simulink model "bh_model_3FB"  (R2023a)
settings: Solver=daessc  StartTime=0.0  StopTime=100  MaxStep=0.005  RelTol=1e-4  AbsTol=1e-4  EnableMultiTasking=on
undefined symbols (not defined in the file or in its folder): env, P0, P1, P2, PA, PB, PC, PG, Points, Springs, Theta, W, X, Y, Z
libraries: sm_lib x34, nesl_utility x17
settings Model: Creator=bhorton  LastModifiedBy=bhorton
settings SolverCC: AutoScaleAbsTol=off  ZeroCrossAlgorithm=Adaptive  AlgebraicLoopSolver=TrustRegion  MaxZcPerStep=1
settings DataIOCC: LimitDataPoints=on  MaxDataPoints=10000  SaveOutput=off  SignalLogging=off  DSMLogging=off  SignalLoggingName=sigout  ReturnWorkspaceOutputsName=SIM_LOG_DATA
settings OptimizationCC: ReuseModelBlockBuffer=off  LifeSpan=inf
settings DebuggingCC: UnconnectedInputMsg=warning  UnconnectedOutputMsg=warning  UnconnectedLineMsg=warning  AllowSymbolicDim=off  SFUnexpectedBacktrackingDiag=warning  SFNoUnconditionalDefaultTransitionDiag=warning  SFExecutionAtInitializationDiag=none  ArithmeticOperatorsInVariantConditions=warning
settings ModelReferenceCC: EnableRefExpFcnMdlSchedulingChecks=on
settings SFSimCC: SimUseLocalCustomCode=off  CustomCodeUndefinedFunction=UseInterfaceOnly
settings RTWCC: RTWUseLocalCustomCode=off  DLArmComputeVersion=19.05
settings CodeAppCC: StateflowObjectComments=on
settings GRTTargetCC: TargetLangStandard=C89/C90 (ANSI)
settings ConfigComp: CovMetricSettings=dw  CovSaveCumulativeToWorkspaceVar=on  CovSaveSingleToWorkspaceVar=on  CovExternalEMLEnable=off  CovSFcnEnable=off
settings SimscapeCC: SimscapeLogType=all  SimscapeLogSimulationStatistics=on  SimscapeLogDataHistory=10000
settings ExplorerConfigSet: InternalSimMechanicsExplorerSettings="<ExplorerConfiguration><canonicalview>default</canonicalview><AnimationSetting><BasePlaybackSpeed>1.0</BasePlaybackSpeed><PlaybackSpeedFactor>1.0</PlaybackSpeedFactor></AnimationSetting><TilePanel><TileInfo><Tiles Columns=\"2\" Count=\"2\" Rows=\"1\"><Column Weight=\"0.4996\"/><Column Weight=\"0.5004\"/><Row Weight=\"1\"/><Tile Height=\"1\" Width=\"1\" X=\"0\" Y=\"0\"/><Tile Height=\"1\" Width=\"1\" X=\"1\" Y=\"0\"/></Tiles></TileInfo><SceneInfo><SceneViewer><BGColor><R>0.60000002384185791</R><G>0.60000002384185791</G><B>0.60000002384185791</B></BGColor><Camera><DoPerspective>off</DoPerspective><Position><X>0.491983639676432549</X><Y>0.660324737193826783</Y><Z>0.997500000159727507</Z></Position><Center><X>0.491983639676432549</X><Y>0.660324737193826783</Y><Z>-0.00249999984027249322</Z></Center><Up><X>0</X><Y>1</Y><Z>-0</Z></Up><ViewLimDist>1</ViewLimDist><YLim>0.930287200234285461</YLim><XLim>0.682141395707506204</XLim></Camera></SceneViewer><SceneViewer><BGColor><R>0.60000002384185791</R><G>0.60000002384185791</G><B>0.60000002384185791</B></BGColor><Camera><DoPerspective>off</DoPerspective><Position><X>0.536343126805734594</X><Y>1.50090638188909886</Y><Z>-0.103056785946452484</Z></Position><Center><X>0.536343126805734594</X><Y>0.499999971795685338</Y><Z>-0.103056785946452484</Z></Center><Up><X>0</X><Y>0</Y><Z>1</Z></Up><ViewLimDist>1</ViewLimDist><YLim>0.956987902738208662</YLim><XLim>0.702787991073371976</XLim></Camera></SceneViewer></SceneInfo></TilePanel><MechEditorPanel><Cameras/><GfxPanelCameraMap/><VideoCreator><PlaybackSpeedRatio>1.0</PlaybackSpeedRatio><FrameRate>30</FrameRate><VideoFormat>Motion JPEG AVI</VideoFormat><FrameSize>auto</FrameSize></VideoCreator></MechEditorPanel></ExplorerConfiguration>"

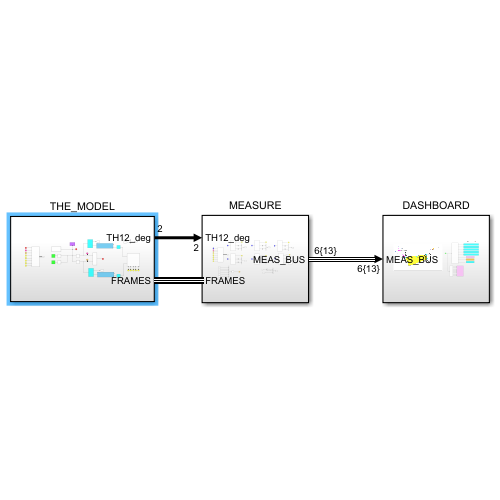
[thumbnail: Simulink's stored preview of the top-level diagram]
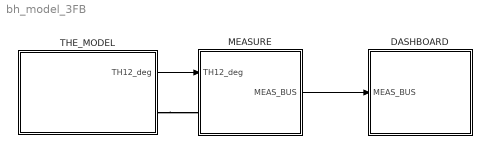
== system bh_model_3FB ==
  DASHBOARD : Subsystem
  MEASURE : Subsystem
  THE_MODEL : Subsystem
      settings: PortSchema="{\"entries\":[{\"content\":{\"sides\":[{\"content\":{\"connectorIds\":[\"Out1\",\"LConn1\"]},\"type\":\"ConnectorPlacement.EquallySpacedRectSide\",\"uuid\":\"a6bd5fb9-d314-4c72-8b76-e48d80fdb19b\"},{\"content\":{\"connectorIds\":[],\"side\":\"RIGHT\"},\"type\":\"ConnectorPlacement.EquallySpacedRectSide\",\"uuid\":\"36a13618-f0d5-425f-9c20-8177aa5c1d72\"},{\"content\":{\"connectorIds\":[],\"side\":\"TOP\"},\"type\":\"ConnectorPlacement.EquallySpacedRectSide\",\"uuid\":\"5c1dc12f-dfae-4687-beb7-ca64844c31e7\"}]},\"type\":\"ConnectorPlacement.EquallySpacedConnector\",\"uuid\":\"dc42e3a7-d8d3-4cef-9db1-f374fadbd399\"}],\"packageUris\":[\"http://schema.mathworks.com/mf0/Connector/R2020b\"],\"version\":\"1.0\"}"
  wires:
  THE_MODEL/1(TH12_deg) -> MEASURE/1(TH12_deg)
  MEASURE/1(MEAS_BUS) -> DASHBOARD/1(MEAS_BUS)
  connections:
  THE_MODEL/LConn1 -- MEASURE/LConn1

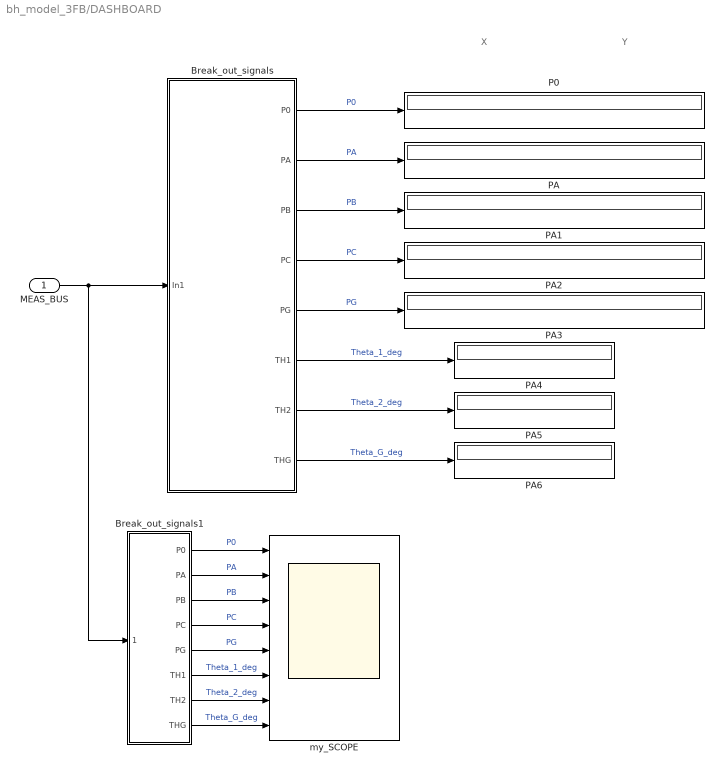
== system bh_model_3FB/DASHBOARD ==
  note: X
  note: Y
  MEAS_BUS : Inport
  Break_out_signals : Subsystem
  Break_out_signals1 : Subsystem
  P0 : Display
  PA{,1..6} (7 alike) : Display
  my_SCOPE : Scope  NumInputPorts=8
  wires:
  MEAS_BUS/1 -> Break_out_signals1/1(MEAS_BUS), Break_out_signals/1(In1)
  Break_out_signals/1(P0) -> P0/1  "P0"
  Break_out_signals/2(PA) -> PA/1  "PA"
  Break_out_signals/3(PB) -> PA1/1  "PB"
  Break_out_signals/4(PC) -> PA2/1  "PC"
  Break_out_signals/5(PG) -> PA3/1  "PG"
  Break_out_signals/6(TH1) -> PA4/1  "Theta_1_deg"
  Break_out_signals/7(TH2) -> PA5/1  "Theta_2_deg"
  Break_out_signals/8(THG) -> PA6/1  "Theta_G_deg"
  Break_out_signals1/1(P0) -> my_SCOPE/1  "P0"
  Break_out_signals1/2(PA) -> my_SCOPE/2  "PA"
  Break_out_signals1/3(PB) -> my_SCOPE/3  "PB"
  Break_out_signals1/4(PC) -> my_SCOPE/4  "PC"
  Break_out_signals1/5(PG) -> my_SCOPE/5  "PG"
  Break_out_signals1/6(TH1) -> my_SCOPE/6  "Theta_1_deg"
  Break_out_signals1/7(TH2) -> my_SCOPE/7  "Theta_2_deg"
  Break_out_signals1/8(THG) -> my_SCOPE/8  "Theta_G_deg"

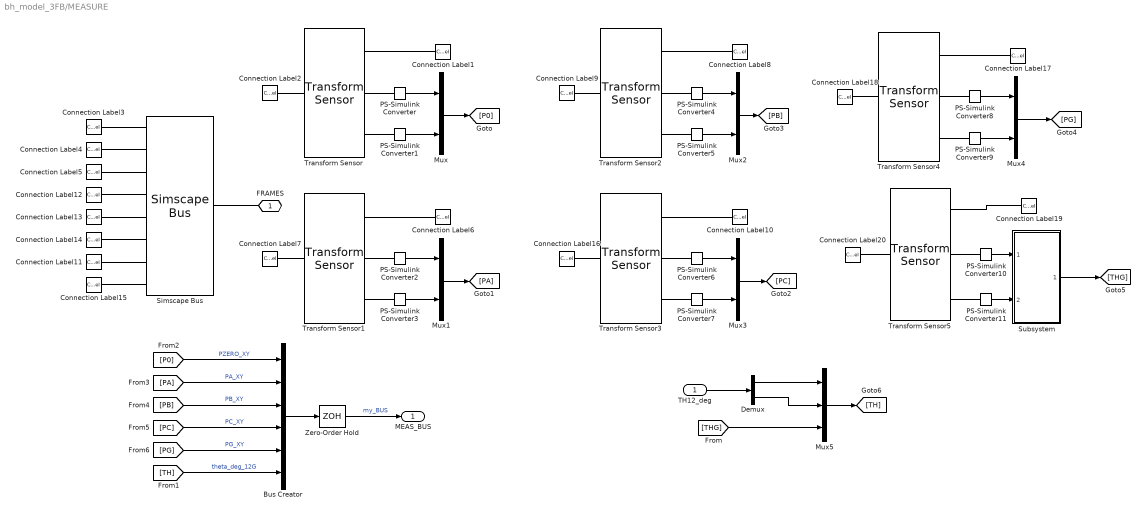
== system bh_model_3FB/MEASURE ==
  TH12_deg : Inport
  Bus Creator : BusCreator  Inputs=6
  Connection Label1 : ConnectionLabel  Label=P0
  Connection Label10 : ConnectionLabel  Label=PC
  Connection Label11 : ConnectionLabel  Label=P0
  Connection Label12 : ConnectionLabel  Label=PA
  Connection Label13 : ConnectionLabel  Label=PB
  Connection Label14 : ConnectionLabel  Label=PC
  Connection Label15 : ConnectionLabel  Label=PG
  Connection Label{2..3,7,9,16,18,20} (7 alike) : ConnectionLabel  Label=W
  Connection Label17 : ConnectionLabel  Label=PG
  Connection Label19 : ConnectionLabel  Label=PG
  Connection Label4 : ConnectionLabel  Label=P1
  Connection Label5 : ConnectionLabel  Label=P2
  Connection Label6 : ConnectionLabel  Label=PA
  Connection Label8 : ConnectionLabel  Label=PB
  Demux : Demux  Outputs=2
  Mux{,1..4} (5 alike) : Mux  Inputs=2
  Mux5 : Mux  Inputs=3
  PS-Simulink Converter{,1..9} (10 alike) : nesl_utility/PS-Simulink Converter  PhysicalDomain=network_engine_domain  SubClassName=ps_output  LeftPortType=input  RightPortType=output  PseudoPeriodic=off  Frequencies=[]  VectorFormat=inherit  Unit=m  AffineConversion=off
  PS-Simulink Converter10 : nesl_utility/PS-Simulink Converter  PhysicalDomain=network_engine_domain  SubClassName=ps_output  LeftPortType=input  RightPortType=output  PseudoPeriodic=off  Frequencies=[]  VectorFormat=inherit  Unit=deg  AffineConversion=off
  PS-Simulink Converter11 : nesl_utility/PS-Simulink Converter  PhysicalDomain=network_engine_domain  SubClassName=ps_output  LeftPortType=input  RightPortType=output  PseudoPeriodic=off  Frequencies=[]  VectorFormat=inherit  Unit=1  AffineConversion=off
  Simscape Bus : SimscapeBus  HierarchyStrings=W;P1;P2;PA;PB;PC;P0;PG
  Subsystem : Subsystem
  Transform Sensor{,1..4} (5 alike) : sm_lib/Frames and Transforms/Transform Sensor  MeasurementFrame=Base  RotationSequence=XYX  SenseAngle=off  SenseAxis=off  SenseQ=off  SenseR=off  SenseRotationSequence=off  SenseOmegaX=off  SenseOmegaY=off  SenseOmegaZ=off  SenseQDot=off  SenseRDot=off  SenseRotationSequenceDot=off  SenseAlphaX=off  SenseAlphaY=off  SenseAlphaZ=off  SenseQDDot=off  SenseRDDot=off  SenseX=on  SenseY=on  SenseZ=off  SenseRad=off  SenseAzim=off  SenseDist=off  SenseInc=off  SenseXDot=off  SenseYDot=off  SenseZDot=off  SenseRadDot=off  SenseAzimDot=off  SenseDistDot=off  SenseIncDot=off  SenseXDDot=off  SenseYDDot=off  SenseZDDot=off  SenseRadDDot=off  SenseAzimDDot=off  SenseDistDDot=off  SenseIncDDot=off
  Transform Sensor5 : sm_lib/Frames and Transforms/Transform Sensor  MeasurementFrame=Base  RotationSequence=XYX  SenseAngle=on  SenseAxis=on  SenseQ=off  SenseR=off  SenseRotationSequence=off  SenseOmegaX=off  SenseOmegaY=off  SenseOmegaZ=off  SenseQDot=off  SenseRDot=off  SenseRotationSequenceDot=off  SenseAlphaX=off  SenseAlphaY=off  SenseAlphaZ=off  SenseQDDot=off  SenseRDDot=off  SenseX=off  SenseY=off  SenseZ=off  SenseRad=off  SenseAzim=off  SenseDist=off  SenseInc=off  SenseXDot=off  SenseYDot=off  SenseZDot=off  SenseRadDot=off  SenseAzimDot=off  SenseDistDot=off  SenseIncDot=off  SenseXDDot=off  SenseYDDot=off  SenseZDDot=off  SenseRadDDot=off  SenseAzimDDot=off  SenseDistDDot=off  SenseIncDDot=off
  Zero-Order Hold : ZeroOrderHold  SampleTime=0.01
  FRAMES : PMIOPort  Side=Left
  MEAS_BUS : Outport
  wires:
  PS-Simulink Converter/1 -> Mux/1
  PS-Simulink Converter1/1 -> Mux/2
  PS-Simulink Converter3/1 -> Mux1/2
  PS-Simulink Converter2/1 -> Mux1/1
  PS-Simulink Converter4/1 -> Mux2/1
  PS-Simulink Converter5/1 -> Mux2/2
  PS-Simulink Converter6/1 -> Mux3/1
  PS-Simulink Converter7/1 -> Mux3/2
  PS-Simulink Converter8/1 -> Mux4/1
  PS-Simulink Converter9/1 -> Mux4/2
  PS-Simulink Converter10/1 -> Subsystem/1(q_deg)
  PS-Simulink Converter11/1 -> Subsystem/2(q_axes)
  Mux/1 -> [P0]
  Mux1/1 -> [PA]
  Mux3/1 -> [PC]
  Mux2/1 -> [PB]
  Mux4/1 -> [PG]
  Subsystem/1(theta_deg) -> [THG]
  TH12_deg/1 -> Demux/1
  Demux/1 -> Mux5/1
  Demux/2 -> Mux5/2
  [THG] -> Mux5/3
  Mux5/1 -> [TH]
  [TH] -> Bus Creator/6  "theta_deg_12G"
  [P0] -> Bus Creator/1  "PZERO_XY"
  [PA] -> Bus Creator/2  "PA_XY"
  [PB] -> Bus Creator/3  "PB_XY"
  [PC] -> Bus Creator/4  "PC_XY"
  [PG] -> Bus Creator/5  "PG_XY"
  Bus Creator/1 -> Zero-Order Hold/1
  Zero-Order Hold/1 -> MEAS_BUS/1  "my_BUS"
  connections:
  Connection Label12/LConn1 -- Simscape Bus/LConn4
  Connection Label13/LConn1 -- Simscape Bus/LConn5
  FRAMES/RConn1 -- Simscape Bus/RConn1
  Connection Label15/LConn1 -- Simscape Bus/LConn8
  Connection Label11/LConn1 -- Simscape Bus/LConn7
  Connection Label4/LConn1 -- Simscape Bus/LConn2
  Connection Label3/LConn1 -- Simscape Bus/LConn1
  Connection Label5/LConn1 -- Simscape Bus/LConn3
  Connection Label14/LConn1 -- Simscape Bus/LConn6
  Connection Label1/LConn1 -- Transform Sensor/RConn1
  PS-Simulink Converter/LConn1 -- Transform Sensor/RConn2
  PS-Simulink Converter1/LConn1 -- Transform Sensor/RConn3
  Connection Label2/LConn1 -- Transform Sensor/LConn1
  Connection Label6/LConn1 -- Transform Sensor1/RConn1
  PS-Simulink Converter2/LConn1 -- Transform Sensor1/RConn2
  PS-Simulink Converter3/LConn1 -- Transform Sensor1/RConn3
  Connection Label7/LConn1 -- Transform Sensor1/LConn1
  Connection Label8/LConn1 -- Transform Sensor2/RConn1
  PS-Simulink Converter5/LConn1 -- Transform Sensor2/RConn3
  Connection Label9/LConn1 -- Transform Sensor2/LConn1
  PS-Simulink Converter4/LConn1 -- Transform Sensor2/RConn2
  PS-Simulink Converter6/LConn1 -- Transform Sensor3/RConn2
  Connection Label10/LConn1 -- Transform Sensor3/RConn1
  PS-Simulink Converter7/LConn1 -- Transform Sensor3/RConn3
  Connection Label16/LConn1 -- Transform Sensor3/LConn1
  PS-Simulink Converter9/LConn1 -- Transform Sensor4/RConn3
  PS-Simulink Converter8/LConn1 -- Transform Sensor4/RConn2
  Connection Label17/LConn1 -- Transform Sensor4/RConn1
  Connection Label18/LConn1 -- Transform Sensor4/LConn1
  Connection Label20/LConn1 -- Transform Sensor5/LConn1
  Connection Label19/LConn1 -- Transform Sensor5/RConn1
  PS-Simulink Converter11/LConn1 -- Transform Sensor5/RConn3
  PS-Simulink Converter10/LConn1 -- Transform Sensor5/RConn2

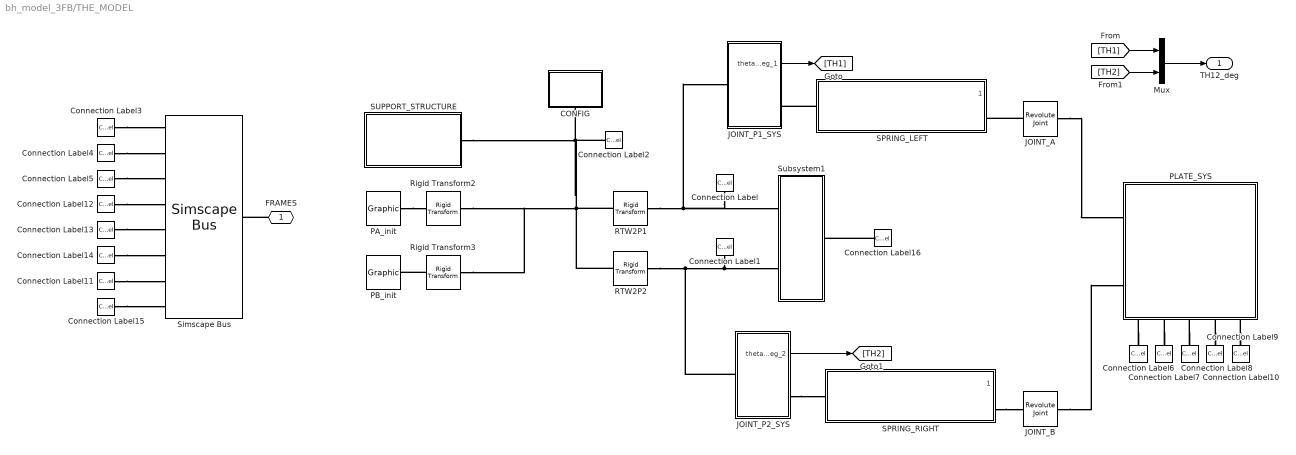
== system bh_model_3FB/THE_MODEL ==
  CONFIG : Subsystem
  Connection Label : ConnectionLabel  Label=P1
  Connection Label1 : ConnectionLabel  Label=P2
  Connection Label10 : ConnectionLabel  Label=P0
  Connection Label11 : ConnectionLabel  Label=P0
  Connection Label12 : ConnectionLabel  Label=PA
  Connection Label13 : ConnectionLabel  Label=PB
  Connection Label14 : ConnectionLabel  Label=PC
  Connection Label15 : ConnectionLabel  Label=PG
  Connection Label16 : ConnectionLabel  Label=W
  Connection Label2 : ConnectionLabel  Label=W
  Connection Label3 : ConnectionLabel  Label=W
  Connection Label4 : ConnectionLabel  Label=P1
  Connection Label5 : ConnectionLabel  Label=P2
  Connection Label6 : ConnectionLabel  Label=PA
  Connection Label7 : ConnectionLabel  Label=PB
  Connection Label8 : ConnectionLabel  Label=PC
  Connection Label9 : ConnectionLabel  Label=PG
  JOINT_A : sm_lib/Joints/Revolute Joint  JointMode=Normal  SenseConstraintForce=off  SenseConstraintForceX=off  SenseConstraintForceY=off  SenseConstraintForceZ=off  SenseConstraintTorque=off  SenseConstraintTorqueX=off  SenseConstraintTorqueY=off  SenseConstraintTorqueZ=off  SenseTotalForce=off  SenseTotalForceX=off  SenseTotalForceY=off  SenseTotalForceZ=off  SenseTotalTorque=off  SenseTotalTorqueX=off  SenseTotalTorqueY=off  SenseTotalTorqueZ=off  CompositeWrenchDir=FollowerOnBase  CompositeWrenchFrame=BaseFrame  EquilibriumPosition=0  EquilibriumPositionUnits=deg  SpringStiffness=0  SpringStiffnessUnits=N*m/deg  DampingCoefficient=0  DampingCoefficientUnits=N*m/(deg/s)  TorqueActuationMode=NoTorque  MotionActuationMode=ComputedMotion  SensePosition=off  SenseVelocity=off  SenseAcceleration=off  SenseTorqueForce=off  SenseLowerLimitTorqueForce=off  SenseUpperLimitTorqueForce=off  LowerLimitSpecify=off  LowerLimitBound=-90  LowerLimitBoundUnits=deg  LowerLimitStiffness=1e4  LowerLimitStiffnessUnits=N*m/deg  LowerLimitDamping=10  LowerLimitDampingUnits=N*m/(deg/s)  LowerLimitTransitionRegionWidth=0.1  LowerLimitTransitionRegionWidthUnits=deg  UpperLimitSpecify=off  UpperLimitBound=90  UpperLimitBoundUnits=deg  UpperLimitStiffness=1e4  UpperLimitStiffnessUnits=N*m/deg  UpperLimitDamping=10  UpperLimitDampingUnits=N*m/(deg/s)  UpperLimitTransitionRegionWidth=0.1  UpperLimitTransitionRegionWidthUnits=deg  PositionTargetSpecify=off  PositionTargetPriority=High  PositionTargetValue=-1*Theta.A_deg  PositionTargetValueUnits=deg  VelocityTargetSpecify=off  VelocityTargetPriority=High  VelocityTargetValue=0  VelocityTargetValueUnits=deg/s
  JOINT_B : sm_lib/Joints/Revolute Joint  JointMode=Normal  SenseConstraintForce=off  SenseConstraintForceX=off  SenseConstraintForceY=off  SenseConstraintForceZ=off  SenseConstraintTorque=off  SenseConstraintTorqueX=off  SenseConstraintTorqueY=off  SenseConstraintTorqueZ=off  SenseTotalForce=off  SenseTotalForceX=off  SenseTotalForceY=off  SenseTotalForceZ=off  SenseTotalTorque=off  SenseTotalTorqueX=off  SenseTotalTorqueY=off  SenseTotalTorqueZ=off  CompositeWrenchDir=FollowerOnBase  CompositeWrenchFrame=BaseFrame  EquilibriumPosition=0  EquilibriumPositionUnits=deg  SpringStiffness=0  SpringStiffnessUnits=N*m/deg  DampingCoefficient=0  DampingCoefficientUnits=N*m/(deg/s)  TorqueActuationMode=NoTorque  MotionActuationMode=ComputedMotion  SensePosition=off  SenseVelocity=off  SenseAcceleration=off  SenseTorqueForce=off  SenseLowerLimitTorqueForce=off  SenseUpperLimitTorqueForce=off  LowerLimitSpecify=off  LowerLimitBound=-90  LowerLimitBoundUnits=deg  LowerLimitStiffness=1e4  LowerLimitStiffnessUnits=N*m/deg  LowerLimitDamping=10  LowerLimitDampingUnits=N*m/(deg/s)  LowerLimitTransitionRegionWidth=0.1  LowerLimitTransitionRegionWidthUnits=deg  UpperLimitSpecify=off  UpperLimitBound=90  UpperLimitBoundUnits=deg  UpperLimitStiffness=1e4  UpperLimitStiffnessUnits=N*m/deg  UpperLimitDamping=10  UpperLimitDampingUnits=N*m/(deg/s)  UpperLimitTransitionRegionWidth=0.1  UpperLimitTransitionRegionWidthUnits=deg  PositionTargetSpecify=off  PositionTargetPriority=High  PositionTargetValue=-1*Theta.B_deg  PositionTargetValueUnits=deg  VelocityTargetSpecify=off  VelocityTargetPriority=High  VelocityTargetValue=0  VelocityTargetValueUnits=deg/s
  JOINT_P1_SYS : Subsystem
  JOINT_P2_SYS : Subsystem
  Mux : Mux  Inputs=2
  PA_init : sm_lib/Body Elements/Graphic  GraphicType=Marker  MarkerShape=Frame  MarkerSize=25  GraphicVisPropType=SimpleVisualProperties  GraphicDiffuseColor=[0 1 0]  GraphicSpecularColor=[0.5 0.5 0.5 1.0]  GraphicAmbientColor=[0.15 0.15 0.15 1.0]  GraphicEmissiveColor=[0.0 0.0 0.0 1.0]  GraphicShininess=75  GraphicOpacity=1.0
  PB_init : sm_lib/Body Elements/Graphic  GraphicType=Marker  MarkerShape=Frame  MarkerSize=25  GraphicVisPropType=SimpleVisualProperties  GraphicDiffuseColor=[0 1 0]  GraphicSpecularColor=[0.5 0.5 0.5 1.0]  GraphicAmbientColor=[0.15 0.15 0.15 1.0]  GraphicEmissiveColor=[0.0 0.0 0.0 1.0]  GraphicShininess=75  GraphicOpacity=1.0
  PLATE_SYS : Subsystem
      settings: PortSchema="{\"entries\":[{\"content\":{\"sides\":[{\"content\":{\"connectorIds\":[\"LConn1\",\"LConn2\"]},\"type\":\"ConnectorPlacement.EquallySpacedRectSide\",\"uuid\":\"93248c55-1ad3-445b-b9a7-56eb06c57406\"},{\"content\":{\"connectorIds\":[],\"side\":\"RIGHT\"},\"type\":\"ConnectorPlacement.EquallySpacedRectSide\",\"uuid\":\"b10a17e2-6726-4405-a35d-9fd4ae8c4b56\"},{\"content\":{\"connectorIds\":[],\"side\":\"TOP\"},\"type\":\"ConnectorPlacement.EquallySpacedRectSide\",\"uuid\":\"5c823850-66f1-4a0f-a96b-d5e6f0dcea4f\"},{\"content\":{\"connectorIds\":[\"RConn1\",\"RConn2\",\"RConn3\",\"RConn4\",\"RConn5\"],\"side\":\"BOTTOM\"},\"type\":\"ConnectorPlacement.EquallySpacedRectSide\",\"uuid\":\"67c94115-9b67-4c68-a1df-5a4847aab27d\"}]},\"type\":\"ConnectorPlacement.EquallySpacedConnector\",\"uuid\":\"0a1a3765-94d9-4f20-8fe4-7302b2902fa4\"}],\"packageUris\":[\"http://schema.mathworks.com/mf0/Connector/R2020b\"],\"version\":\"1.0\"}"
  RTW2P1 : sm_lib/Frames and Transforms/Rigid Transform  TranslationMethod=Cartesian  TranslationStandardOffset=0  TranslationStandardOffsetUnits=m  TranslationStandardAxis=+Z  TranslationCartesianOffset=[Points.P1, 0]  TranslationCartesianOffsetUnits=m  TranslationROffset=0  TranslationROffsetUnits=m  TranslationZOffset=0  TranslationZOffsetUnits=m  TranslationThetaOffset=0  TranslationThetaOffsetUnits=deg  RotationMethod=None  RotationAngleUnits=deg  RotationStandardAxis=+Z  RotationAngle=0.0  RotationArbitraryAxis=[0 0 1]  FollAlignAxisA=+X  BaseAlignAxisA=+Y  FollAlignAxisB=+Y  BaseAlignAxisB=+Z  RotationSequenceAxes=FollowerAxes  RotationSequence=XYX  RotationSequenceAngles=[0 0 0]  RotationSequenceAnglesUnits=deg  RotationMatrix=[1 0 0; 0 1 0; 0 0 1]  Quaternion=[1 0 0 0]
  RTW2P2 : sm_lib/Frames and Transforms/Rigid Transform  TranslationMethod=Cartesian  TranslationStandardOffset=0  TranslationStandardOffsetUnits=m  TranslationStandardAxis=+Z  TranslationCartesianOffset=[Points.P2, 0]  TranslationCartesianOffsetUnits=m  TranslationROffset=0  TranslationROffsetUnits=m  TranslationZOffset=0  TranslationZOffsetUnits=m  TranslationThetaOffset=0  TranslationThetaOffsetUnits=deg  RotationMethod=None  RotationAngleUnits=deg  RotationStandardAxis=+Z  RotationAngle=0.0  RotationArbitraryAxis=[0 0 1]  FollAlignAxisA=+X  BaseAlignAxisA=+Y  FollAlignAxisB=+Y  BaseAlignAxisB=+Z  RotationSequenceAxes=FollowerAxes  RotationSequence=XYX  RotationSequenceAngles=[0 0 0]  RotationSequenceAnglesUnits=deg  RotationMatrix=[1 0 0; 0 1 0; 0 0 1]  Quaternion=[1 0 0 0]
  Rigid Transform2 : sm_lib/Frames and Transforms/Rigid Transform  TranslationMethod=Cartesian  TranslationStandardOffset=0  TranslationStandardOffsetUnits=m  TranslationStandardAxis=+Z  TranslationCartesianOffset=[Points.PA, 0]  TranslationCartesianOffsetUnits=m  TranslationROffset=0  TranslationROffsetUnits=m  TranslationZOffset=0  TranslationZOffsetUnits=m  TranslationThetaOffset=0  TranslationThetaOffsetUnits=deg  RotationMethod=None  RotationAngleUnits=deg  RotationStandardAxis=+Z  RotationAngle=0.0  RotationArbitraryAxis=[0 0 1]  FollAlignAxisA=+X  BaseAlignAxisA=+Y  FollAlignAxisB=+Y  BaseAlignAxisB=+Z  RotationSequenceAxes=FollowerAxes  RotationSequence=XYX  RotationSequenceAngles=[0 0 0]  RotationSequenceAnglesUnits=deg  RotationMatrix=[1 0 0; 0 1 0; 0 0 1]  Quaternion=[1 0 0 0]
  Rigid Transform3 : sm_lib/Frames and Transforms/Rigid Transform  TranslationMethod=Cartesian  TranslationStandardOffset=0  TranslationStandardOffsetUnits=m  TranslationStandardAxis=+Z  TranslationCartesianOffset=[Points.PB, 0]  TranslationCartesianOffsetUnits=m  TranslationROffset=0  TranslationROffsetUnits=m  TranslationZOffset=0  TranslationZOffsetUnits=m  TranslationThetaOffset=0  TranslationThetaOffsetUnits=deg  RotationMethod=None  RotationAngleUnits=deg  RotationStandardAxis=+Z  RotationAngle=0.0  RotationArbitraryAxis=[0 0 1]  FollAlignAxisA=+X  BaseAlignAxisA=+Y  FollAlignAxisB=+Y  BaseAlignAxisB=+Z  RotationSequenceAxes=FollowerAxes  RotationSequence=XYX  RotationSequenceAngles=[0 0 0]  RotationSequenceAnglesUnits=deg  RotationMatrix=[1 0 0; 0 1 0; 0 0 1]  Quaternion=[1 0 0 0]
  SPRING_LEFT : Subsystem  ReferencedSubsystem=bh_COMPONENT_spring_SYS  k=Springs.LEFT.stiffness  c=Springs.LEFT.damping  EQ_L=Springs.LEFT.free_length  tip_pos_L=Springs.LEFT.initial_length  VIS_L=Springs.LEFT.visual_length  VIS_R=Springs.LEFT.visual_R
  SPRING_RIGHT : Subsystem  ReferencedSubsystem=bh_COMPONENT_spring_SYS  k=Springs.RIGHT.stiffness  c=Springs.RIGHT.damping  EQ_L=Springs.RIGHT.free_length  tip_pos_L=Springs.RIGHT.initial_length  VIS_L=Springs.RIGHT.visual_length  VIS_R=Springs.RIGHT.visual_R
  SUPPORT_STRUCTURE : Subsystem
  Simscape Bus : SimscapeBus  HierarchyStrings=W;P1;P2;PA;PB;PC;P0;PG
  Subsystem1 : Subsystem
  FRAMES : PMIOPort  Side=Left
  TH12_deg : Outport
  wires:
  JOINT_P2_SYS/1(theta_deg_2) -> [TH2]
  JOINT_P1_SYS/1(theta_deg_1) -> [TH1]
  [TH1] -> Mux/1
  [TH2] -> Mux/2
  Mux/1 -> TH12_deg/1
  connections:
  Connection Label15/LConn1 -- Simscape Bus/LConn8
  Connection Label11/LConn1 -- Simscape Bus/LConn7
  FRAMES/RConn1 -- Simscape Bus/RConn1
  RTW2P2/LConn1 -- RTW2P1/LConn1 -- Rigid Transform3/LConn1 -- Rigid Transform2/LConn1 -- Connection Label2/LConn1 -- SUPPORT_STRUCTURE/LConn1 -- CONFIG/LConn1
  PA_init/RConn1 -- Rigid Transform2/RConn1
  JOINT_B/RConn1 -- PLATE_SYS/LConn2
  Connection Label4/LConn1 -- Simscape Bus/LConn2
  Connection Label9/LConn1 -- PLATE_SYS/RConn4
  Connection Label10/LConn1 -- PLATE_SYS/RConn5
  Rigid Transform3/RConn1 -- PB_init/RConn1
  Connection Label5/LConn1 -- Simscape Bus/LConn3
  JOINT_A/RConn1 -- PLATE_SYS/LConn1
  Connection Label7/LConn1 -- PLATE_SYS/RConn2
  Connection Label14/LConn1 -- Simscape Bus/LConn6
  Connection Label6/LConn1 -- PLATE_SYS/RConn1
  Connection Label8/LConn1 -- PLATE_SYS/RConn3
  Connection Label12/LConn1 -- Simscape Bus/LConn4
  Connection Label3/LConn1 -- Simscape Bus/LConn1
  JOINT_A/LConn1 -- SPRING_LEFT/RConn1
  Connection Label13/LConn1 -- Simscape Bus/LConn5
  Connection Label/LConn1 -- Subsystem1/RConn1 -- RTW2P1/RConn1 -- JOINT_P1_SYS/LConn1
  JOINT_P2_SYS/LConn1 -- Connection Label1/LConn1 -- Subsystem1/RConn2 -- RTW2P2/RConn1
  Connection Label16/LConn1 -- Subsystem1/LConn1
  SPRING_LEFT/LConn1 -- JOINT_P1_SYS/RConn1
  JOINT_P2_SYS/RConn1 -- SPRING_RIGHT/LConn1
  SPRING_RIGHT/RConn1 -- JOINT_B/LConn1

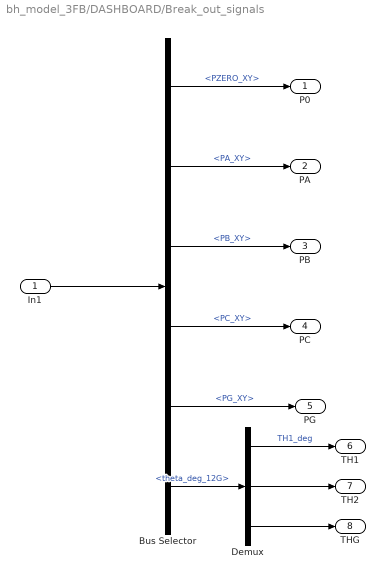
== system bh_model_3FB/DASHBOARD/Break_out_signals ==
  In1 : Inport
  Bus Selector : BusSelector  OutputSignals=PZERO_XY,PA_XY,PB_XY,PC_XY,PG_XY,theta_deg_12G
  Demux : Demux  Outputs=3
  P0 : Outport
  PA : Outport  Port=2
  PB : Outport  Port=3
  PC : Outport  Port=4
  PG : Outport  Port=5
  TH1 : Outport  Port=6
  TH2 : Outport  Port=7
  THG : Outport  Port=8
  wires:
  Demux/3 -> THG/1
  Bus Selector/3 -> PB/1  "<PB_XY>"
  Bus Selector/2 -> PA/1  "<PA_XY>"
  Bus Selector/5 -> PG/1  "<PG_XY>"
  Demux/1 -> TH1/1  "TH1_deg"
  Demux/2 -> TH2/1
  Bus Selector/6 -> Demux/1  "<theta_deg_12G>"
  Bus Selector/4 -> PC/1  "<PC_XY>"
  Bus Selector/1 -> P0/1  "<PZERO_XY>"
  In1/1 -> Bus Selector/1

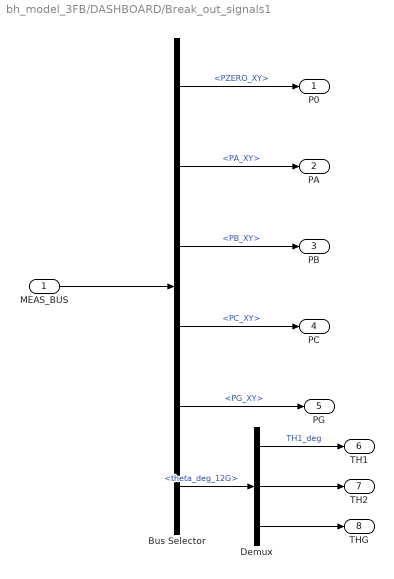
== system bh_model_3FB/DASHBOARD/Break_out_signals1 ==
  MEAS_BUS : Inport
  Bus Selector : BusSelector  OutputSignals=PZERO_XY,PA_XY,PB_XY,PC_XY,PG_XY,theta_deg_12G
  Demux : Demux  Outputs=3
  P0 : Outport
  PA : Outport  Port=2
  PB : Outport  Port=3
  PC : Outport  Port=4
  PG : Outport  Port=5
  TH1 : Outport  Port=6
  TH2 : Outport  Port=7
  THG : Outport  Port=8
  wires:
  Demux/3 -> THG/1
  Bus Selector/3 -> PB/1  "<PB_XY>"
  Bus Selector/2 -> PA/1  "<PA_XY>"
  Bus Selector/5 -> PG/1  "<PG_XY>"
  Demux/1 -> TH1/1  "TH1_deg"
  Demux/2 -> TH2/1
  Bus Selector/6 -> Demux/1  "<theta_deg_12G>"
  Bus Selector/4 -> PC/1  "<PC_XY>"
  Bus Selector/1 -> P0/1  "<PZERO_XY>"
  MEAS_BUS/1 -> Bus Selector/1

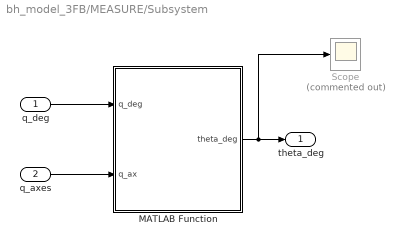
== system bh_model_3FB/MEASURE/Subsystem ==
  q_deg : Inport
  q_axes : Inport  Port=2
  MATLAB Function : MATLAB Function  TreatAsAtomicUnit=on
  Scope : Scope  Commented=on
  theta_deg : Outport
  wires:
  q_deg/1 -> MATLAB Function/1(q_deg)
  q_axes/1 -> MATLAB Function/2(q_ax)
  MATLAB Function/1(theta_deg) -> Scope/1, theta_deg/1

== system bh_model_3FB/THE_MODEL/CONFIG ==
  Mechanism Configuration : sm_lib/Utilities/Mechanism Configuration  UniformGravity=Constant  GravityVector=[0, -1*env.g, 0]  GravityVectorUnits=m/s^2  LinearizationDelta=0.001  JointModeTransitionNonlinearIterations=2
  Solver Configuration : nesl_utility/Solver Configuration  PhysicalDomain=network_engine_domain  SubClassName=solver  LeftPortType=input  RightPortType=generic  Tones=[]  Harmonics=[]  SimulateNoise=off  Profile=off  UseLocalSampling=off  EnableSwitchedLinearOptims=on  FrequencyDomain=off  UseCCode=off  RelTol=0.001  AbsTol=1e-06  MinStep=1e-09  ToWorkspace=off  RevertToSquareIcSolve=off  NumHomotopyIterations=100  PhasorMode=off  PhasorModeNumHarmonics=1  ConsistencySolver=NEWTON_FTOL  IndexReductionMethod=DerivativeReplacement  DoDC=off  ResidualTolerance=1e-09  ConsistencyTolSource=GLOBAL  ConsistencyAbsTol=0.001  ConsistencyRelTol=0.001  ConsistencyTolFactor=0.001  UseLocalSolver=off  LocalSolverChoice=NE_BACKWARD_EULER_ADVANCER  ResolveIndetEquations=on  FunctionEvalNumThread=1  LocalSolverSampleTime=0.001  DoFixedCost=off  MaxNonlinIter=3  MaxModeIter=2  ComputeImpulses=off  ImpulseIterations=2  LinearAlgebra=Sparse  LinearAlgebraNumThread=0  EquationFormulation=NE_TIME_EF  DelaysMemoryBudget=1024  AutomaticFiltering=on  FilteringTimeConstant=0.001  PartitionStorageMethod=AS_NEEDED  PartitionMemoryBudget=1024  PartitionMethod=FAST
  World Frame : sm_lib/Frames and Transforms/World Frame
  W : PMIOPort  Side=Left
  connections:
  World Frame/RConn1 -- Solver Configuration/RConn1 -- W/RConn1 -- Mechanism Configuration/RConn1

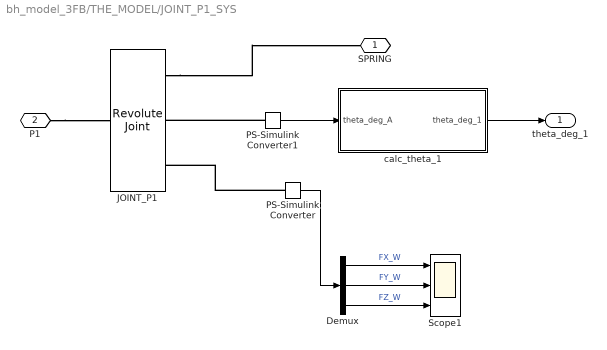
== system bh_model_3FB/THE_MODEL/JOINT_P1_SYS ==
  Demux : Demux  Outputs=3
  JOINT_P1 : sm_lib/Joints/Revolute Joint  JointMode=Normal  SenseConstraintForce=on  SenseConstraintForceX=off  SenseConstraintForceY=off  SenseConstraintForceZ=off  SenseConstraintTorque=off  SenseConstraintTorqueX=off  SenseConstraintTorqueY=off  SenseConstraintTorqueZ=off  SenseTotalForce=off  SenseTotalForceX=off  SenseTotalForceY=off  SenseTotalForceZ=off  SenseTotalTorque=off  SenseTotalTorqueX=off  SenseTotalTorqueY=off  SenseTotalTorqueZ=off  CompositeWrenchDir=BaseOnFollower  CompositeWrenchFrame=BaseFrame  EquilibriumPosition=0  EquilibriumPositionUnits=deg  SpringStiffness=0  SpringStiffnessUnits=N*m/deg  DampingCoefficient=0  DampingCoefficientUnits=N*m/(deg/s)  TorqueActuationMode=NoTorque  MotionActuationMode=ComputedMotion  SensePosition=on  SenseVelocity=off  SenseAcceleration=off  SenseTorqueForce=off  SenseLowerLimitTorqueForce=off  SenseUpperLimitTorqueForce=off  LowerLimitSpecify=off  LowerLimitBound=-90  LowerLimitBoundUnits=deg  LowerLimitStiffness=1e4  LowerLimitStiffnessUnits=N*m/deg  LowerLimitDamping=10  LowerLimitDampingUnits=N*m/(deg/s)  LowerLimitTransitionRegionWidth=0.1  LowerLimitTransitionRegionWidthUnits=deg  UpperLimitSpecify=off  UpperLimitBound=90  UpperLimitBoundUnits=deg  UpperLimitStiffness=1e4  UpperLimitStiffnessUnits=N*m/deg  UpperLimitDamping=10  UpperLimitDampingUnits=N*m/(deg/s)  UpperLimitTransitionRegionWidth=0.1  UpperLimitTransitionRegionWidthUnits=deg  PositionTargetSpecify=on  PositionTargetPriority=High  PositionTargetValue=Theta.A_deg  PositionTargetValueUnits=deg  VelocityTargetSpecify=on  VelocityTargetPriority=High  VelocityTargetValue=0  VelocityTargetValueUnits=deg/s
  PS-Simulink Converter : nesl_utility/PS-Simulink Converter  PhysicalDomain=network_engine_domain  SubClassName=ps_output  LeftPortType=input  RightPortType=output  PseudoPeriodic=off  Frequencies=[]  VectorFormat=inherit  Unit=N  AffineConversion=off
  PS-Simulink Converter1 : nesl_utility/PS-Simulink Converter  PhysicalDomain=network_engine_domain  SubClassName=ps_output  LeftPortType=input  RightPortType=output  PseudoPeriodic=off  Frequencies=[]  VectorFormat=inherit  Unit=deg  AffineConversion=off
  Scope1 : Scope  NumInputPorts=3
  calc_theta_1 : Subsystem
  SPRING : PMIOPort  Side=Right
  P1 : PMIOPort  Port=2  Side=Left
  theta_deg_1 : Outport
  wires:
  Demux/2 -> Scope1/2  "FY_W"
  PS-Simulink Converter/1 -> Demux/1
  Demux/1 -> Scope1/1  "FX_W"
  Demux/3 -> Scope1/3  "FZ_W"
  PS-Simulink Converter1/1 -> calc_theta_1/1(theta_deg_A)
  calc_theta_1/1(theta_deg_1) -> theta_deg_1/1
  connections:
  JOINT_P1/RConn1 -- SPRING/RConn1
  P1/RConn1 -- JOINT_P1/LConn1
  PS-Simulink Converter/LConn1 -- JOINT_P1/RConn3
  PS-Simulink Converter1/LConn1 -- JOINT_P1/RConn2

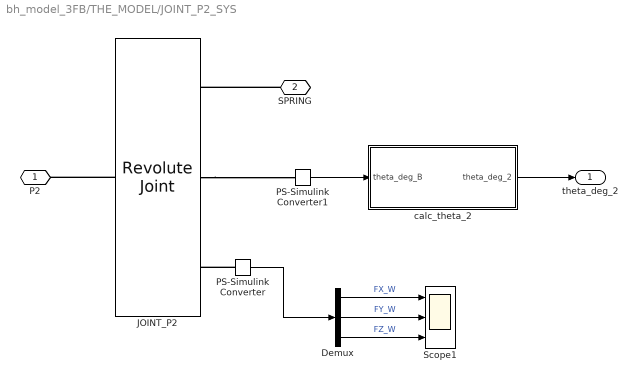
== system bh_model_3FB/THE_MODEL/JOINT_P2_SYS ==
  Demux : Demux  Outputs=3
  JOINT_P2 : sm_lib/Joints/Revolute Joint  JointMode=Normal  SenseConstraintForce=on  SenseConstraintForceX=off  SenseConstraintForceY=off  SenseConstraintForceZ=off  SenseConstraintTorque=off  SenseConstraintTorqueX=off  SenseConstraintTorqueY=off  SenseConstraintTorqueZ=off  SenseTotalForce=off  SenseTotalForceX=off  SenseTotalForceY=off  SenseTotalForceZ=off  SenseTotalTorque=off  SenseTotalTorqueX=off  SenseTotalTorqueY=off  SenseTotalTorqueZ=off  CompositeWrenchDir=FollowerOnBase  CompositeWrenchFrame=BaseFrame  EquilibriumPosition=0  EquilibriumPositionUnits=deg  SpringStiffness=0  SpringStiffnessUnits=N*m/deg  DampingCoefficient=0  DampingCoefficientUnits=N*m/(deg/s)  TorqueActuationMode=NoTorque  MotionActuationMode=ComputedMotion  SensePosition=on  SenseVelocity=off  SenseAcceleration=off  SenseTorqueForce=off  SenseLowerLimitTorqueForce=off  SenseUpperLimitTorqueForce=off  LowerLimitSpecify=off  LowerLimitBound=-90  LowerLimitBoundUnits=deg  LowerLimitStiffness=1e4  LowerLimitStiffnessUnits=N*m/deg  LowerLimitDamping=10  LowerLimitDampingUnits=N*m/(deg/s)  LowerLimitTransitionRegionWidth=0.1  LowerLimitTransitionRegionWidthUnits=deg  UpperLimitSpecify=off  UpperLimitBound=90  UpperLimitBoundUnits=deg  UpperLimitStiffness=1e4  UpperLimitStiffnessUnits=N*m/deg  UpperLimitDamping=10  UpperLimitDampingUnits=N*m/(deg/s)  UpperLimitTransitionRegionWidth=0.1  UpperLimitTransitionRegionWidthUnits=deg  PositionTargetSpecify=on  PositionTargetPriority=High  PositionTargetValue=Theta.B_deg  PositionTargetValueUnits=deg  VelocityTargetSpecify=on  VelocityTargetPriority=High  VelocityTargetValue=0  VelocityTargetValueUnits=deg/s
  PS-Simulink Converter : nesl_utility/PS-Simulink Converter  PhysicalDomain=network_engine_domain  SubClassName=ps_output  LeftPortType=input  RightPortType=output  PseudoPeriodic=off  Frequencies=[]  VectorFormat=inherit  Unit=N  AffineConversion=off
  PS-Simulink Converter1 : nesl_utility/PS-Simulink Converter  PhysicalDomain=network_engine_domain  SubClassName=ps_output  LeftPortType=input  RightPortType=output  PseudoPeriodic=off  Frequencies=[]  VectorFormat=inherit  Unit=deg  AffineConversion=off
  Scope1 : Scope  NumInputPorts=3
  calc_theta_2 : Subsystem
  P2 : PMIOPort  Side=Left
  SPRING : PMIOPort  Port=2  Side=Right
  theta_deg_2 : Outport
  wires:
  Demux/1 -> Scope1/1  "FX_W"
  Demux/3 -> Scope1/3  "FZ_W"
  Demux/2 -> Scope1/2  "FY_W"
  PS-Simulink Converter/1 -> Demux/1
  calc_theta_2/1(theta_deg_2) -> theta_deg_2/1
  PS-Simulink Converter1/1 -> calc_theta_2/1(theta_deg_B)
  connections:
  JOINT_P2/LConn1 -- P2/RConn1
  SPRING/RConn1 -- JOINT_P2/RConn1
  PS-Simulink Converter/LConn1 -- JOINT_P2/RConn3
  JOINT_P2/RConn2 -- PS-Simulink Converter1/LConn1

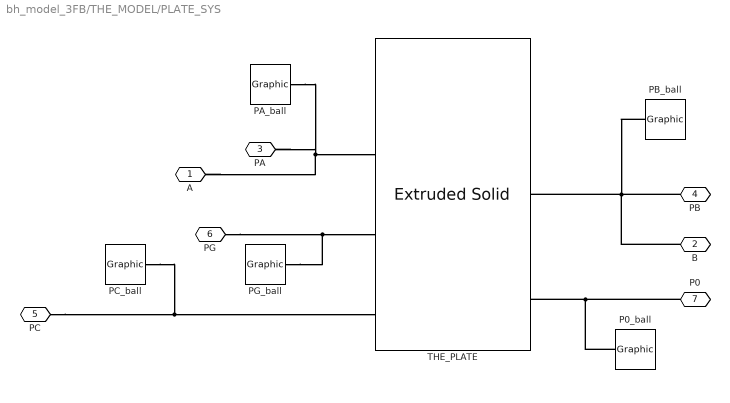
== system bh_model_3FB/THE_MODEL/PLATE_SYS ==
  P0_ball : sm_lib/Body Elements/Graphic  GraphicType=Marker  MarkerShape=Sphere  MarkerSize=10  GraphicVisPropType=SimpleVisualProperties  GraphicDiffuseColor=[0 1 1]  GraphicSpecularColor=[0.5 0.5 0.5 1.0]  GraphicAmbientColor=[0.15 0.15 0.15 1.0]  GraphicEmissiveColor=[0.0 0.0 0.0 1.0]  GraphicShininess=75  GraphicOpacity=1.0
  PA_ball : sm_lib/Body Elements/Graphic  GraphicType=Marker  MarkerShape=Sphere  MarkerSize=10  GraphicVisPropType=SimpleVisualProperties  GraphicDiffuseColor=[0 1 1]  GraphicSpecularColor=[0.5 0.5 0.5 1.0]  GraphicAmbientColor=[0.15 0.15 0.15 1.0]  GraphicEmissiveColor=[0.0 0.0 0.0 1.0]  GraphicShininess=75  GraphicOpacity=1.0
  PB_ball : sm_lib/Body Elements/Graphic  GraphicType=Marker  MarkerShape=Sphere  MarkerSize=10  GraphicVisPropType=SimpleVisualProperties  GraphicDiffuseColor=[0 1 1]  GraphicSpecularColor=[0.5 0.5 0.5 1.0]  GraphicAmbientColor=[0.15 0.15 0.15 1.0]  GraphicEmissiveColor=[0.0 0.0 0.0 1.0]  GraphicShininess=75  GraphicOpacity=1.0
  PC_ball : sm_lib/Body Elements/Graphic  GraphicType=Marker  MarkerShape=Sphere  MarkerSize=10  GraphicVisPropType=SimpleVisualProperties  GraphicDiffuseColor=[0 1 1]  GraphicSpecularColor=[0.5 0.5 0.5 1.0]  GraphicAmbientColor=[0.15 0.15 0.15 1.0]  GraphicEmissiveColor=[0.0 0.0 0.0 1.0]  GraphicShininess=75  GraphicOpacity=1.0
  PG_ball : sm_lib/Body Elements/Graphic  GraphicType=Marker  MarkerShape=Sphere  MarkerSize=10  GraphicVisPropType=SimpleVisualProperties  GraphicDiffuseColor=[0 1 1]  GraphicSpecularColor=[0.5 0.5 0.5 1.0]  GraphicAmbientColor=[0.15 0.15 0.15 1.0]  GraphicEmissiveColor=[0.0 0.0 0.0 1.0]  GraphicShininess=75  GraphicOpacity=1.0
  THE_PLATE : sm_lib/Body Elements/Extruded Solid  GraphicAmbientColor=[0.15 0.15 0.15 1.0]  BasedOnType=Density  CenterOfMass=[0 0 0]  CenterOfMassUnits=m  GraphicDiffuseColor=[1.0 1.0 0.0]  ExportConvexHullGeometry=off  ExtrusionCrossSection=quad_obj.get_xy  ExtrusionCrossSectionUnits=m  Density=quad_obj.density  DensityUnits=kg/m^3  DoExposeReferenceFrame=on  GraphicEmissiveColor=[0.0 0.0 0.0 1.0]  ExportEntireGeometry=off  ExtrusionLength=quad_obj.z_thick  ExtrusionLengthUnits=m  ExtrusionType=General  SerializedFrames=<Frames><Frame><Id>Frame1</Id><Value><Name>CoM</Name><Origin><Source>CenterOfMassFrame</Source><FeatureName></FeatureName></Origin><PrimaryAxis><DefinedDirection>+Z</DefinedDirection><Source>ReferenceFrame</Source><SourceDirection>+Z</SourceDirection><FeatureName></FeatureName></PrimaryAxis><SecondaryAxis><DefinedDirection>+X</DefinedDirection><Source>ReferenceFrame</Source><SourceDirection>+X</SourceDirection><FeatureName></FeatureName></SecondaryAxis></Value></Frame><Frame><Id>Frame2</Id><Value><Name>A</Name><Origin><Source>GeometricFeature</Source><FeatureName>top point 4</FeatureName></Origin><PrimaryAxis><DefinedDirection>+Z</DefinedDirection><Source>ReferenceFrame</Source><SourceDirection>+Z</SourceDirection><FeatureName></FeatureName></PrimaryAxis><SecondaryAxis><DefinedDirection>+X</DefinedDirection><Source>ReferenceFrame</Source><SourceDirection>+X</SourceDirection><FeatureName></FeatureName></SecondaryAxis></Value></Frame><Frame><Id>Frame3</Id><Value><Name>B</Name><Origin><Source>GeometricFeature</Source><FeatureName>top point 3</FeatureName></Origin><PrimaryAxis><DefinedDirection>+Z</DefinedDirection><Source>ReferenceFrame</Source><SourceDirection>+Z</SourceDirection><FeatureName></FeatureName></PrimaryAxis><SecondaryAxis><DefinedDirection>+X</DefinedDirection><Source>ReferenceFrame</Source><SourceDirection>+X</SourceDirection><FeatureName></FeatureName></SecondaryAxis></Value></Frame><Frame><Id>Frame4</Id><Value><Name>COM_face</Name><Origin><Source>GeometricFeature</Source><FeatureName>top surface</FeatureName></Origin><PrimaryAxis><DefinedDirection>+Z</DefinedDirection><Source>ReferenceFrame</Source><SourceDirection>+Z</SourceDirection><FeatureName></FeatureName></PrimaryAxis><SecondaryAxis><DefinedDirection>+X</DefinedDirection><Source>ReferenceFrame</Source><SourceDirection>+X</SourceDirection><FeatureName></FeatureName></SecondaryAxis></Value></Frame><Frame><Id>Frame5</Id><Value><Name>0</Name><Origin><Source>GeometricFeature</Source><FeatureName>top point 1</FeatureName></Origin><PrimaryAxis><DefinedDirection>+Z</DefinedDirection><Source>ReferenceFrame</Source><SourceDirection>+Z</SourceDirection><FeatureName></FeatureName></PrimaryAxis><SecondaryAxis><DefinedDirection>+X</DefinedDirection><Source>ReferenceFrame</Source><SourceDirection>+X</SourceDirection><FeatureName></FeatureName></SecondaryAxis></Value></Frame><Frame><Id>Frame6</Id><Value><Name>C</Name><Origin><Source>GeometricFeature</Source><FeatureName>top point 2</FeatureName></Origin><PrimaryAxis><DefinedDirection>+Z</DefinedDirection><Source>ReferenceFrame</Source><SourceDirection>+Z</SourceDirection><FeatureName></FeatureName></PrimaryAxis><SecondaryAxis><DefinedDirection>+X</DefinedDirection><Source>ReferenceFrame</Source><SourceDirection>+X</SourceDirection><FeatureName></FeatureName></SecondaryAxis></Value></Frame></Frames>  MarkerShape=Sphere  MarkerSize=10  GraphicType=FromGeometry  InertiaType=CalculateFromGeometry  Mass=1  MassUnits=kg  MomentsOfInertia=[1 1 1]  MomentsOfInertiaUnits=kg*m^2  PolygonNumSides=3  GraphicOpacity=1.0  PolygonOuterRadius=1  PolygonOuterRadiusUnits=m  ProductsOfInertia=[0 0 0]  ProductsOfInertiaUnits=kg*m^2  GraphicShininess=75  GraphicSpecularColor=[0.5 0.5 0.5 1.0]  GraphicVisPropType=SimpleVisualProperties
  A : PMIOPort  Side=Left
  B : PMIOPort  Port=2  Side=Left
  PA : PMIOPort  Port=3  Side=Right
  PB : PMIOPort  Port=4  Side=Right
  PC : PMIOPort  Port=5  Side=Right
  PG : PMIOPort  Port=6  Side=Right
  P0 : PMIOPort  Port=7  Side=Right
  connections:
  B/RConn1 -- PB_ball/RConn1 -- PB/RConn1 -- THE_PLATE/RConn2
  A/RConn1 -- PA_ball/RConn1 -- PA/RConn1 -- THE_PLATE/LConn2
  PG/RConn1 -- PG_ball/RConn1 -- THE_PLATE/LConn3
  PC/RConn1 -- THE_PLATE/LConn4 -- PC_ball/RConn1
  P0/RConn1 -- P0_ball/RConn1 -- THE_PLATE/RConn3

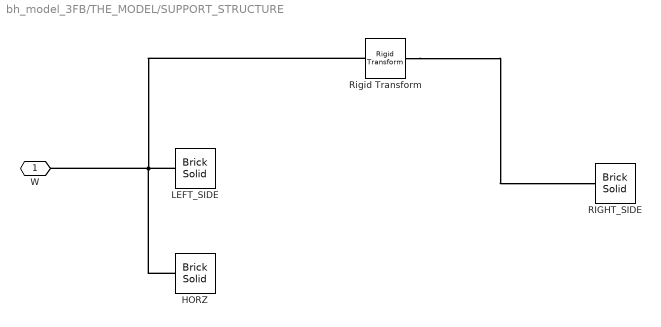
== system bh_model_3FB/THE_MODEL/SUPPORT_STRUCTURE ==
  HORZ : sm_lib/Body Elements/Brick Solid  GraphicAmbientColor=[0.15 0.15 0.15 1.0]  BasedOnType=Density  BrickDimensions=Support.HORZ.dims  BrickDimensionsUnits=m  CenterOfMass=[0 0 0]  CenterOfMassUnits=m  GraphicDiffuseColor=[0.0 0.0 0.0]  Density=1000  DensityUnits=kg/m^3  DoExposeReferenceFrame=on  GraphicEmissiveColor=[0.0 0.0 0.0 1.0]  ExportEntireGeometry=off  SerializedFrames=<Frames><Frame><Id>Frame1</Id><Value><Name>0</Name><Origin><Source>GeometricFeature</Source><FeatureName>+z -x curve</FeatureName></Origin><PrimaryAxis><DefinedDirection>+Z</DefinedDirection><Source>ReferenceFrame</Source><SourceDirection>+Z</SourceDirection><FeatureName></FeatureName></PrimaryAxis><SecondaryAxis><DefinedDirection>+X</DefinedDirection><Source>ReferenceFrame</Source><SourceDirection>+X</SourceDirection><FeatureName></FeatureName></SecondaryAxis></Value></Frame></Frames>  MarkerShape=Sphere  MarkerSize=10  GraphicType=FromGeometry  InertiaType=CalculateFromGeometry  Mass=1  MassUnits=kg  MomentsOfInertia=[1 1 1]  MomentsOfInertiaUnits=kg*m^2  GraphicOpacity=1.0  ProductsOfInertia=[0 0 0]  ProductsOfInertiaUnits=kg*m^2  GraphicShininess=75  GraphicSpecularColor=[0.5 0.5 0.5 1.0]  GraphicVisPropType=SimpleVisualProperties
  LEFT_SIDE : sm_lib/Body Elements/Brick Solid  GraphicAmbientColor=[0.15 0.15 0.15 1.0]  BasedOnType=Density  BrickDimensions=Support.VERT.dims  BrickDimensionsUnits=m  CenterOfMass=[0 0 0]  CenterOfMassUnits=m  GraphicDiffuseColor=[0.0 0.0 0.0]  Density=1000  DensityUnits=kg/m^3  DoExposeReferenceFrame=on  GraphicEmissiveColor=[0.0 0.0 0.0 1.0]  ExportEntireGeometry=off  SerializedFrames=<Frames><Frame><Id>Frame1</Id><Value><Name>0</Name><Origin><Source>GeometricFeature</Source><FeatureName>-y +z curve</FeatureName></Origin><PrimaryAxis><DefinedDirection>+Z</DefinedDirection><Source>ReferenceFrame</Source><SourceDirection>+Z</SourceDirection><FeatureName></FeatureName></PrimaryAxis><SecondaryAxis><DefinedDirection>+X</DefinedDirection><Source>ReferenceFrame</Source><SourceDirection>+X</SourceDirection><FeatureName></FeatureName></SecondaryAxis></Value></Frame></Frames>  MarkerShape=Sphere  MarkerSize=10  GraphicType=FromGeometry  InertiaType=CalculateFromGeometry  Mass=1  MassUnits=kg  MomentsOfInertia=[1 1 1]  MomentsOfInertiaUnits=kg*m^2  GraphicOpacity=1.0  ProductsOfInertia=[0 0 0]  ProductsOfInertiaUnits=kg*m^2  GraphicShininess=75  GraphicSpecularColor=[0.5 0.5 0.5 1.0]  GraphicVisPropType=SimpleVisualProperties
  RIGHT_SIDE : sm_lib/Body Elements/Brick Solid  GraphicAmbientColor=[0.15 0.15 0.15 1.0]  BasedOnType=Density  BrickDimensions=Support.VERT.dims  BrickDimensionsUnits=m  CenterOfMass=[0 0 0]  CenterOfMassUnits=m  GraphicDiffuseColor=[0.0 0.0 0.0]  Density=1000  DensityUnits=kg/m^3  DoExposeReferenceFrame=on  GraphicEmissiveColor=[0.0 0.0 0.0 1.0]  ExportEntireGeometry=off  SerializedFrames=<Frames><Frame><Id>Frame1</Id><Value><Name>0</Name><Origin><Source>GeometricFeature</Source><FeatureName>-y +z curve</FeatureName></Origin><PrimaryAxis><DefinedDirection>+Z</DefinedDirection><Source>ReferenceFrame</Source><SourceDirection>+Z</SourceDirection><FeatureName></FeatureName></PrimaryAxis><SecondaryAxis><DefinedDirection>+X</DefinedDirection><Source>ReferenceFrame</Source><SourceDirection>+X</SourceDirection><FeatureName></FeatureName></SecondaryAxis></Value></Frame></Frames>  MarkerShape=Sphere  MarkerSize=10  GraphicType=FromGeometry  InertiaType=CalculateFromGeometry  Mass=1  MassUnits=kg  MomentsOfInertia=[1 1 1]  MomentsOfInertiaUnits=kg*m^2  GraphicOpacity=1.0  ProductsOfInertia=[0 0 0]  ProductsOfInertiaUnits=kg*m^2  GraphicShininess=75  GraphicSpecularColor=[0.5 0.5 0.5 1.0]  GraphicVisPropType=SimpleVisualProperties
  Rigid Transform : sm_lib/Frames and Transforms/Rigid Transform  TranslationMethod=StandardAxis  TranslationStandardOffset=Points.P2(1)-Points.P1(1)  TranslationStandardOffsetUnits=m  TranslationStandardAxis=+X  TranslationCartesianOffset=[0 0 0]  TranslationCartesianOffsetUnits=m  TranslationROffset=0  TranslationROffsetUnits=m  TranslationZOffset=0  TranslationZOffsetUnits=m  TranslationThetaOffset=0  TranslationThetaOffsetUnits=deg  RotationMethod=None  RotationAngleUnits=deg  RotationStandardAxis=+Z  RotationAngle=0.0  RotationArbitraryAxis=[0 0 1]  FollAlignAxisA=+X  BaseAlignAxisA=+Y  FollAlignAxisB=+Y  BaseAlignAxisB=+Z  RotationSequenceAxes=FollowerAxes  RotationSequence=XYX  RotationSequenceAngles=[0 0 0]  RotationSequenceAnglesUnits=deg  RotationMatrix=[1 0 0; 0 1 0; 0 0 1]  Quaternion=[1 0 0 0]
  W : PMIOPort  Side=Left
  connections:
  LEFT_SIDE/LConn1 -- W/RConn1 -- Rigid Transform/LConn1 -- HORZ/LConn1
  Rigid Transform/RConn1 -- RIGHT_SIDE/LConn1

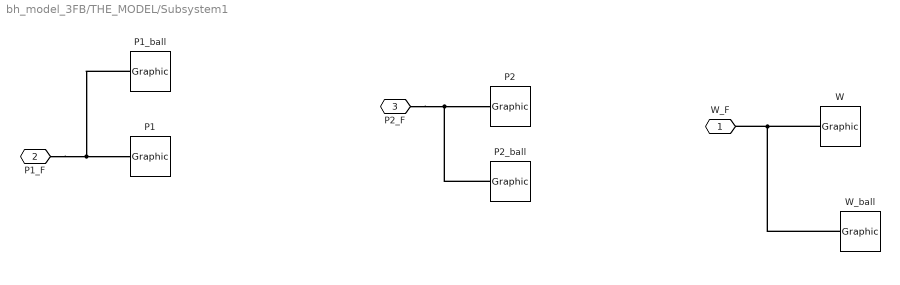
== system bh_model_3FB/THE_MODEL/Subsystem1 ==
  P1 : sm_lib/Body Elements/Graphic  GraphicType=Marker  MarkerShape=Frame  MarkerSize=45  GraphicVisPropType=SimpleVisualProperties  GraphicDiffuseColor=[1 0.07451 0.651]  GraphicSpecularColor=[0.5 0.5 0.5 1.0]  GraphicAmbientColor=[0.15 0.15 0.15 1.0]  GraphicEmissiveColor=[0.0 0.0 0.0 1.0]  GraphicShininess=75  GraphicOpacity=1.0
  P1_ball : sm_lib/Body Elements/Graphic  GraphicType=Marker  MarkerShape=Sphere  MarkerSize=20  GraphicVisPropType=SimpleVisualProperties  GraphicDiffuseColor=[1 0.07451 0.651]  GraphicSpecularColor=[0.5 0.5 0.5 1.0]  GraphicAmbientColor=[0.15 0.15 0.15 1.0]  GraphicEmissiveColor=[0.0 0.0 0.0 1.0]  GraphicShininess=75  GraphicOpacity=1.0
  P2 : sm_lib/Body Elements/Graphic  GraphicType=Marker  MarkerShape=Frame  MarkerSize=45  GraphicVisPropType=SimpleVisualProperties  GraphicDiffuseColor=[0.9294 0.6941 0.1255]  GraphicSpecularColor=[0.5 0.5 0.5 1.0]  GraphicAmbientColor=[0.15 0.15 0.15 1.0]  GraphicEmissiveColor=[0.0 0.0 0.0 1.0]  GraphicShininess=75  GraphicOpacity=1.0
  P2_ball : sm_lib/Body Elements/Graphic  GraphicType=Marker  MarkerShape=Sphere  MarkerSize=20  GraphicVisPropType=SimpleVisualProperties  GraphicDiffuseColor=[0.9294 0.6941 0.1255]  GraphicSpecularColor=[0.5 0.5 0.5 1.0]  GraphicAmbientColor=[0.15 0.15 0.15 1.0]  GraphicEmissiveColor=[0.0 0.0 0.0 1.0]  GraphicShininess=75  GraphicOpacity=1.0
  W : sm_lib/Body Elements/Graphic  GraphicType=Marker  MarkerShape=Frame  MarkerSize=60  GraphicVisPropType=SimpleVisualProperties  GraphicDiffuseColor=[1 0 0]  GraphicSpecularColor=[0.5 0.5 0.5 1.0]  GraphicAmbientColor=[0.15 0.15 0.15 1.0]  GraphicEmissiveColor=[0.0 0.0 0.0 1.0]  GraphicShininess=75  GraphicOpacity=1.0
  W_ball : sm_lib/Body Elements/Graphic  GraphicType=Marker  MarkerShape=Sphere  MarkerSize=30  GraphicVisPropType=SimpleVisualProperties  GraphicDiffuseColor=[1 0 0]  GraphicSpecularColor=[0.5 0.5 0.5 1.0]  GraphicAmbientColor=[0.15 0.15 0.15 1.0]  GraphicEmissiveColor=[0.0 0.0 0.0 1.0]  GraphicShininess=75  GraphicOpacity=1.0
  W_F : PMIOPort  Side=Left
  P1_F : PMIOPort  Port=2  Side=Right
  P2_F : PMIOPort  Port=3  Side=Right
  connections:
  P2_F/RConn1 -- P2_ball/RConn1 -- P2/RConn1
  P1_F/RConn1 -- P1_ball/RConn1 -- P1/RConn1
  W/RConn1 -- W_ball/RConn1 -- W_F/RConn1

== system bh_model_3FB/THE_MODEL/JOINT_P1_SYS/calc_theta_1 ==
  theta_deg_A : Inport
  Gain : Gain  Gain=-1
  Scope : Scope
  theta_deg_1 : Outport
  wires:
  theta_deg_A/1 -> Gain/1
  Gain/1 -> Scope/1, theta_deg_1/1

== system bh_model_3FB/THE_MODEL/JOINT_P2_SYS/calc_theta_2 ==
  theta_deg_B : Inport
  MATLAB Function : MATLAB Function  TreatAsAtomicUnit=on
  Scope : Scope
  theta_deg_2 : Outport
  wires:
  theta_deg_B/1 -> MATLAB Function/1(theta_deg_B)
  MATLAB Function/1(theta_deg_2) -> Scope/1, theta_deg_2/1

== matlab function bh_model_3FB/MEASURE/Subsystem/MATLAB Function ==
  data: q_deg input; theta_deg output; q_ax input
function theta_deg = fcn(q_deg, q_ax)

    if(q_ax(3) < 0)
        theta_deg = -1 * q_deg;
    else
        theta_deg =      q_deg;
    end

end

== matlab function bh_model_3FB/THE_MODEL/JOINT_P2_SYS/calc_theta_2/MATLAB Function ==
  data: theta_deg_B input; theta_deg_2 output
function theta_deg_2 = fcn(theta_deg_B)

    if(theta_deg_B > 0 )
         theta_deg_2    = theta_deg_B - 180;
    else
          theta_deg_2   = 180  + theta_deg_B;
    end

end
